simulink model "lowpassfliter"  (R2024a)
settings: Solver=FixedStepAuto  StartTime=0.0  StopTime=10.0  FixedStep=1e-5  RelTol=1e-3
libraries: mcbcontrolslib x2, simulink x1
settings Model: Creator=wsl  LastModifiedBy=wsl

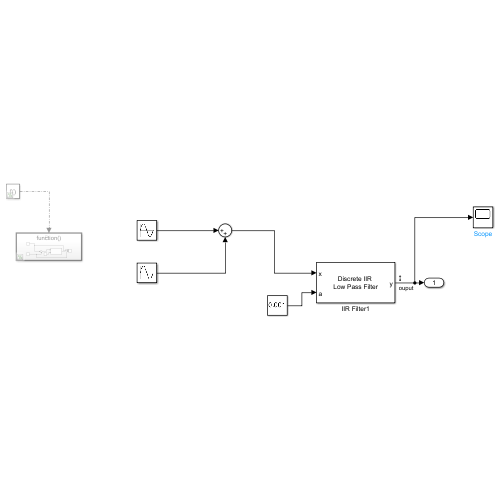
[thumbnail: Simulink's stored preview of the top-level diagram]
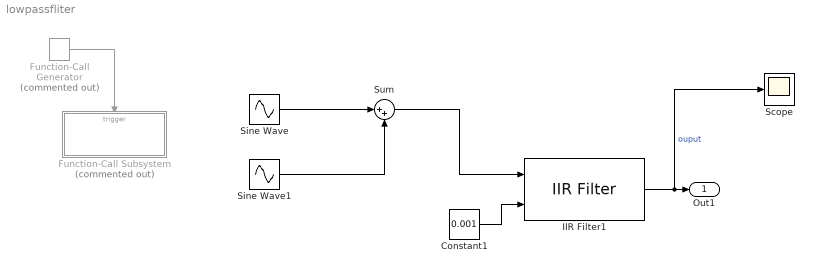
== system lowpassfliter ==
  Constant1 : Constant  Value=0.001
  Function-Call Generator : simulink/Ports & Subsystems/Function-Call Generator  Commented=on  sample_time=1e-5  numberOfIterations=1  DisallowWideOutput=off
  Function-Call Subsystem : Subsystem  Commented=on  TreatAsAtomicUnit=on
  IIR Filter1 : mcbcontrolslib/IIR Filter  VariantControl=Low Pass Filter  VariantSelect=Low-pass  FilterConstantInputType=Input port  Filter_constant=0.01  advancedSettings=off  Ts=50e-6  cutOff_freq=32.1525
      settings: LibrarySourceBlock=mcblib/Signal Management/IIR Filter
  Scope : Scope
  Sine Wave : Sin  Frequency=20*pi
  Sine Wave1 : Sin  Frequency=40*pi
  Sum : Sum  Inputs=|++
  Out1 : Outport
  wires:
  Function-Call Generator/1 -> Function-Call Subsystem/Trigger
  IIR Filter1/1 -> Scope/1, Out1/1  "ouput"
  Sum/1 -> IIR Filter1/1
  Constant1/1 -> IIR Filter1/2
  Sine Wave/1 -> Sum/1
  Sine Wave1/1 -> Sum/2

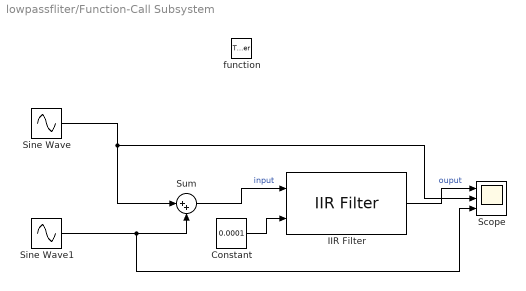
== system lowpassfliter/Function-Call Subsystem ==
  function : TriggerPort  TriggerType=function-call  VariantControl=(inherit)
  Constant : Constant  Value=0.0001
  IIR Filter : mcbcontrolslib/IIR Filter  VariantControl=Low Pass Filter  VariantSelect=Low-pass  FilterConstantInputType=Input port  Filter_constant=0.01  advancedSettings=off  Ts=50e-6  cutOff_freq=32.1525
      settings: LibrarySourceBlock=mcblib/Signal Management/IIR Filter
  Scope : Scope  NumInputPorts=3
  Sine Wave : Sin  Frequency=2*pi
  Sine Wave1 : Sin  Frequency=2000*pi
  Sum : Sum  Inputs=|++
  wires:
  Sine Wave/1 -> Scope/2, Sum/1
  Sine Wave1/1 -> Scope/3, Sum/2
  Sum/1 -> IIR Filter/1  "input"
  IIR Filter/1 -> Scope/1  "ouput"
  Constant/1 -> IIR Filter/2
